simulink model "motor_model"  (R2018b)
settings: Solver=VariableStepAuto  StartTime=0.0  StopTime=1  RelTol=1e-3
InitFcn:
  | motor_parameters
values from neighbouring files (symbols this model uses):
  b = 0.5    [motor_parameters.m]
  J = 12e-9    (= 1.2e-08)    [motor_model_new.m]    (also in motor_parameters.m = 0.01)
  K = 0.025    [motor_parameters.m]
  L = 2.3e-3    (= 0.0023)    [motor_model_new.m]    (also in motor_parameters.m = 0.05)
  R = eye(3) .* 1e-6    [KalmanFilter.m]    (also in model.m = 1; model_2link.m = 1; motor_model_new.m = 2.18; motor_parameters.m = 2)
libraries: powerlib x7, simulink x1, pePwmGenerator x1
settings Model: Creator=sasrinivas  LastModifiedBy=sasrinivas
settings SolverCC: ZeroCrossAlgorithm=Adaptive
settings DebuggingCC: IgnoredZcDiagnostic=none

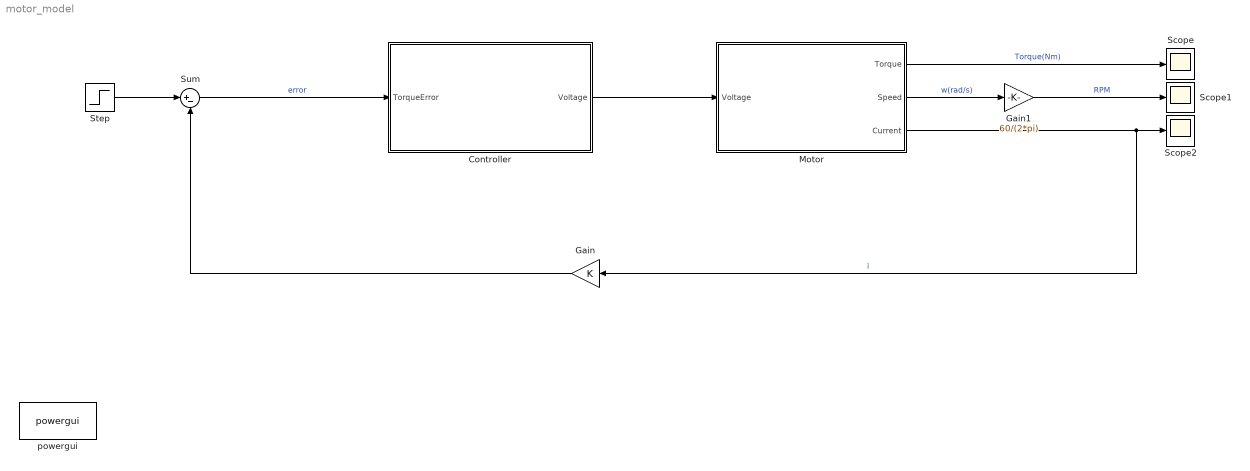
== system motor_model ==
  Controller : Subsystem
  Gain : Gain  Gain=K
  Gain1 : Gain  Gain=60/(2*pi)
  Motor : Subsystem
  Scope : Scope
  Scope1 : Scope
  Scope2 : Scope
  Step : Step  Time=0.5  Before=0.01  After=0.03  SampleTime=0
  Sum : Sum  Inputs=|+-
  powergui : powerlib/powergui  Priority=1  SimulationMode=Continuous  SampleTime=50e-6  frequency=60  Iterations=50  frequencyindice=0  Pbase=100e6  ErrMax=1e-4  UnitsV=kV  UnitsW=MW  buscounter=0  FunctionMessages=off  echomessages=off  EnableUseOfTLC=off  CurrentSourceSwitches=off  DisableSnubberDevices=off  DisableRonSwitches=off  DisableVfSwitches=off  DisplayEquations=off  SolverType=Tustin/Backward Euler (TBE)  Interpol=off  ExternalGateDelay=off  methode=off  Ts=100  x0status=blocks  SPID=on  SwTol=0  HookPort=off  RestoreLinks=warning  ResistiveCurrentMeasurement=off  Frange=[0:2:500]  Ylog=off  Xlog=on  ShowGrid=off  save=off  variable=ZData  structure=0  ZoomFFT=off  StartTime=0.0  cycles=1  DisplayStyle=1  fundamental=60  FreqAxis=off  MaxFrequency=1000  frequencyindicesteady=1  RmsSteady=1  display=off
  wires:
  Motor/1(Torque) -> Scope/1  "Torque(Nm)"
  Motor/2(Speed) -> Gain1/1  "w(rad/s)"
  Motor/3(Current) -> Gain/1, Scope2/1  "i"
  Controller/1(Voltage) -> Motor/1(Voltage)
  Step/1 -> Sum/1
  Gain/1 -> Sum/2
  Sum/1 -> Controller/1(TorqueError)  "error"
  Gain1/1 -> Scope1/1  "RPM"

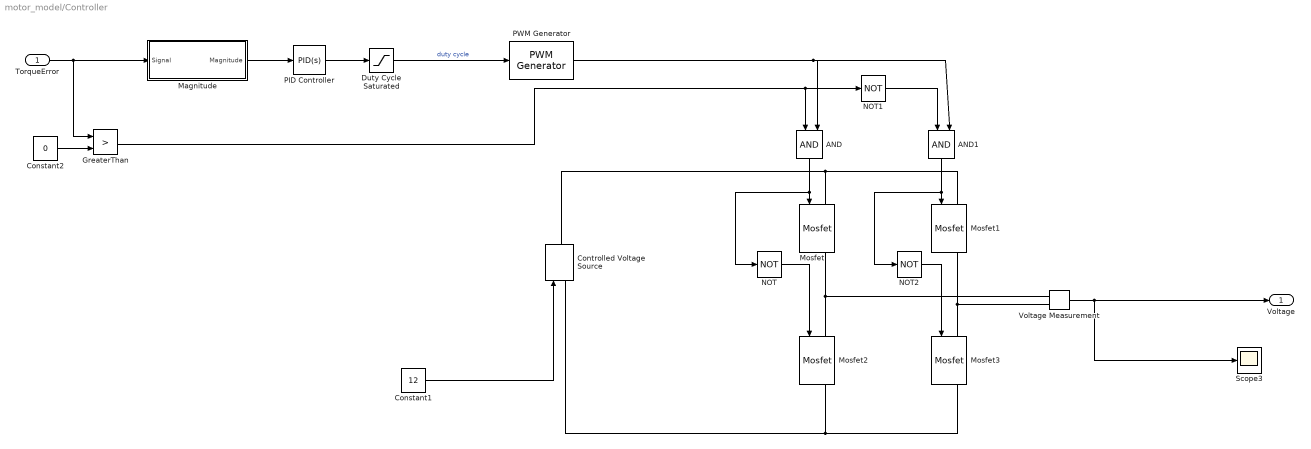
== system motor_model/Controller ==
  TorqueError : Inport
  AND : Logic  IconShape=distinctive  AllPortsSameDT=off  OutDataTypeStr=boolean
  AND1 : Logic  IconShape=distinctive  AllPortsSameDT=off  OutDataTypeStr=boolean
  Constant1 : Constant  Value=12
  Constant2 : Constant  Value=0
  Controlled Voltage Source : powerlib/Electrical Sources/Controlled Voltage Source  Initialize=on  Source_Type=DC  Amplitude=0  Phase=0  Frequency=0  Measurements=None
  Duty Cycle Saturated : Saturate  UpperLimit=0.95  LowerLimit=0.01
  GreaterThan : RelationalOperator  Operator=>  OutDataTypeStr=boolean  RndMeth=Simplest
  Magnitude : Subsystem
  Mosfet{,1..3} (4 alike) : powerlib/Power Electronics/Mosfet  Ron=0.01  Lon=0  Rd=0.01  Vfd=0  IC=0  Rs=1e5  Cs=inf  Measurements=on
  NOT : Logic  Operator=NOT  IconShape=distinctive  AllPortsSameDT=off  OutDataTypeStr=boolean
  NOT1 : Logic  Operator=NOT  IconShape=distinctive  AllPortsSameDT=off  OutDataTypeStr=boolean
  NOT2 : Logic  Operator=NOT  IconShape=distinctive  AllPortsSameDT=off  OutDataTypeStr=boolean
  PID Controller : simulink/Continuous/PID Controller  Controller=PID  Form=Parallel  TimeDomain=Continuous-time  SampleTime=-1  IntegratorMethod=Forward Euler  FilterMethod=Forward Euler  ControllerParametersSource=internal  P=20.3  I=1456.13  D=0.004  UseFilter=on  N=100  TunerSelectOption=Transfer Function Based (PID Tuner App)  InitialConditionSource=internal  InitialConditionForIntegrator=0  InitialConditionForFilter=0  DifferentiatorICPrevScaledInput=0  ExternalReset=none  TrackingMode=off  Kt=1  LimitOutput=off  UpperSaturationLimit=inf  LowerSaturationLimit=-inf  LinearizeAsGain=on  AntiWindupMode=none  Kb=1  POutMin=[]  POutMax=[]  IOutMin=[]  IOutMax=[]  DOutMin=[]  DOutMax=[]  NOutMin=[]  NOutMax=[]  SumOutMin=[]  SumOutMax=[]  SaturationOutMin=[]  SaturationOutMax=[]  PParamMin=[]  PParamMax=[]  IParamMin=[]  IParamMax=[]  DParamMin=[]  DParamMax=[]  NParamMin=[]  NParamMax=[]  KbParamMin=[]  KbParamMax=[]  KtParamMin=[]  KtParamMax=[]  KbOutMin=[]  KbOutMax=[]  KtOutMin=[]  KtOutMax=[]  IntegratorOutMin=[]  IntegratorOutMax=[]  FilterOutMin=[]  FilterOutMax=[]  SumI1OutMin=[]  SumI1OutMax=[]  SumI2OutMin=[]  SumI2OutMax=[]  SumI3OutMin=[]  SumI3OutMax=[]  SumI4OutMin=[]  SumI4OutMax=[]  SumDOutMin=[]  SumDOutMax=[]  DifferentiatorOutMin=[]  DifferentiatorOutMax=[]  FilterDiffOutCoefMin=[]  FilterDiffOutCoefMax=[]  ReciprocalOutMin=[]  ReciprocalOutMax=[]  SumDenOutMin=[]  SumDenOutMax=[]  SumNumOutMin=[]  SumNumOutMax=[]  DivideOutMin=[]  DivideOutMax=[]  IntegratorContinuousStateAttributes=''  IntegratorStateMustResolveToSignalObject=off  IntegratorRTWStateStorageClass=Auto  FilterContinuousStateAttributes=''  FilterStateMustResolveToSignalObject=off  FilterRTWStateStorageClass=Auto  ParallelPVariant=InternalParameters  IdealPVariant=Disabled  IVariant=InternalParameters  DVariant=InternalParameters  IntegratorVariant=Continuous  SatVariant=Disabled  AWVariant=Passthrough  PCopyVariant=Disabled  TRVariant=Disabled  FdbkBlocksVariant=Forward  IdealPFdbkVariant=Disabled  SatFdbkVariant=Disabled  DerivativeFilterVariant=ContFilter  NVariant=InternalParameters  NCopyVariant=Disabled  FilterICVariant=InternalICsFilter  IntegratorICVariant=InternalICs  ExternalResetVariant=Disabled  TRSumVariant=Passthrough  SumFdbkVariant=Disabled  SumVariant=Sum_PID
  PWM Generator : pePwmGenerator/PWM Generator  CarrCount=Up  Tper=1e-3  Ts=5e-5
  Scope3 : Scope
  Voltage Measurement : powerlib/Measurements/Voltage Measurement  PhasorSimulation=off  OutputType=Complex  PSBequivalent=0
  Voltage : Outport
  wires:
  Constant1/1 -> Controlled Voltage Source/1
  NOT/1 -> Mosfet2/1
  PWM Generator/1 -> AND/2, AND1/2
  AND/1 -> NOT/1, Mosfet/1
  AND1/1 -> NOT2/1, Mosfet1/1
  NOT1/1 -> AND1/1
  NOT2/1 -> Mosfet3/1
  TorqueError/1 -> Magnitude/1(Signal), GreaterThan/1
  Magnitude/1(Magnitude) -> PID Controller/1
  Constant2/1 -> GreaterThan/2
  GreaterThan/1 -> AND/1, NOT1/1
  Voltage Measurement/1 -> Scope3/1, Voltage/1
  PID Controller/1 -> Duty Cycle Saturated/1
  Duty Cycle Saturated/1 -> PWM Generator/1  "duty cycle"
  connections:
  Controlled Voltage Source/LConn1 -- Mosfet2/RConn1 -- Mosfet3/RConn1
  Controlled Voltage Source/RConn1 -- Mosfet1/LConn1 -- Mosfet/LConn1
  Mosfet/RConn1 -- Mosfet2/LConn1 -- Voltage Measurement/LConn1
  Mosfet1/RConn1 -- Voltage Measurement/LConn2 -- Mosfet3/LConn1

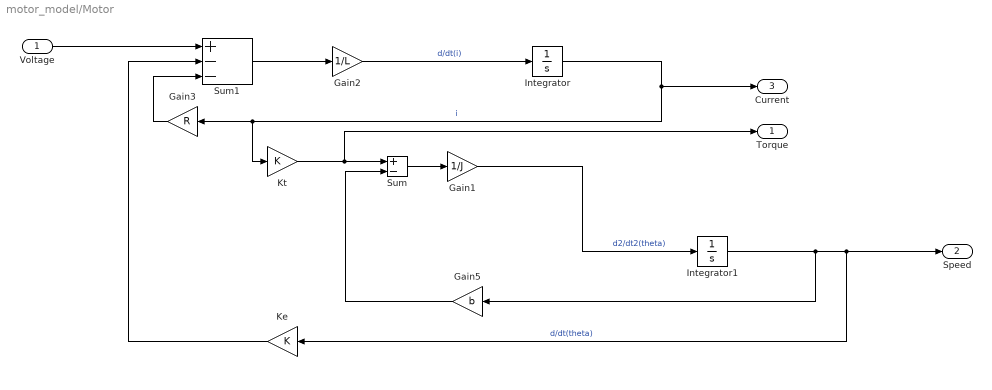
== system motor_model/Motor ==
  Voltage : Inport
  Gain1 : Gain  Gain=1/J
  Gain2 : Gain  Gain=1/L
  Gain3 : Gain  Gain=R
  Gain5 : Gain  Gain=b
  Integrator : Integrator
  Integrator1 : Integrator
  Ke : Gain  Gain=K
  Kt : Gain  Gain=K
  Sum : Sum  Inputs=+-
  Sum1 : Sum  Inputs=+--
  Torque : Outport
  Speed : Outport  Port=2
  Current : Outport  Port=3
  wires:
  Sum/1 -> Gain1/1
  Integrator1/1 -> Gain5/1, Speed/1, Ke/1  "d/dt(theta)"
  Integrator/1 -> Current/1, Kt/1, Gain3/1  "i"
  Gain1/1 -> Integrator1/1  "d2/dt2(theta)"
  Ke/1 -> Sum1/2
  Gain3/1 -> Sum1/3
  Sum1/1 -> Gain2/1
  Gain2/1 -> Integrator/1  "d/dt(i)"
  Kt/1 -> Torque/1, Sum/1
  Voltage/1 -> Sum1/1
  Gain5/1 -> Sum/2

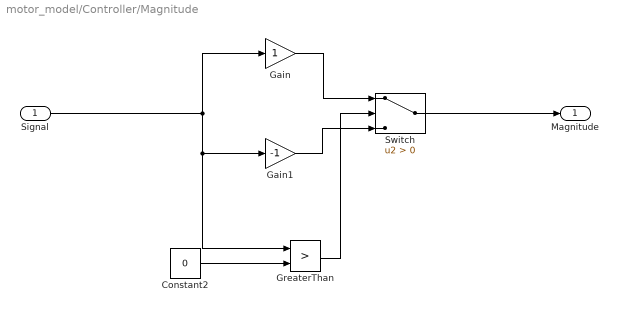
== system motor_model/Controller/Magnitude ==
  Signal : Inport
  Constant2 : Constant  Value=0
  Gain : Gain
  Gain1 : Gain  Gain=-1
  GreaterThan : RelationalOperator  Operator=>  OutDataTypeStr=boolean  RndMeth=Simplest
  Switch : Switch  Criteria=u2 > Threshold
  Magnitude : Outport
  wires:
  Signal/1 -> Gain/1, Gain1/1, GreaterThan/1
  Gain/1 -> Switch/1
  GreaterThan/1 -> Switch/2
  Constant2/1 -> GreaterThan/2
  Gain1/1 -> Switch/3
  Switch/1 -> Magnitude/1
